simulink model "untitled2"  (R2016a)
settings: Solver=VariableStepAuto  StartTime=0.0  StopTime=500  FixedStep=0.01  RelTol=1e-3
undefined symbols (not defined in the file or in its folder): ref_speed
libraries: simulink x1
settings Model: Creator=91968  LastModifiedBy=91968

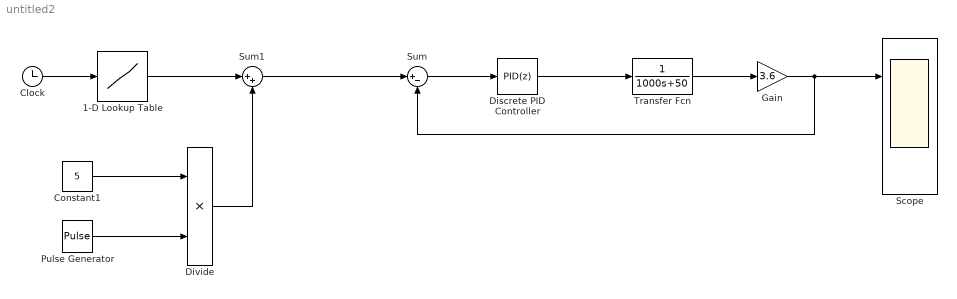
== system untitled2 ==
  1-D Lookup Table : Lookup_n-D  NumberOfTableDimensions=1  BreakpointsForDimension1=[-5:5]  Table=ref_speed(1:500)  InternalRulePriority=Speed  RndMeth=Simplest  InputSameDT=on
  Clock : Clock
  Constant1 : Constant  Value=5  VectorParams1D=off
  Discrete PID Controller : simulink/Continuous/PID Controller  Controller=PID  TimeDomain=Discrete-time  SampleTime=1  IntegratorMethod=Forward Euler  FilterMethod=Forward Euler  Form=Parallel  UseFilter=on  ControllerParametersSource=internal  P=200  I=7.1  D=0  N=100  InitialConditionSource=internal  InitialConditionForIntegrator=0  InitialConditionForFilter=0  ExternalReset=none  LimitOutput=on  UpperSaturationLimit=4200  LowerSaturationLimit=-inf  LinearizeAsGain=off  AntiWindupMode=none  Kb=1  TrackingMode=off  Kt=1  PParamMin=[]  PParamMax=[]  IParamMin=[]  IParamMax=[]  DParamMin=[]  DParamMax=[]  NParamMin=[]  NParamMax=[]  KbParamMin=[]  KbParamMax=[]  KtParamMin=[]  KtParamMax=[]  POutMin=[]  POutMax=[]  IOutMin=[]  IOutMax=[]  DOutMin=[]  DOutMax=[]  NOutMin=[]  NOutMax=[]  KbOutMin=[]  KbOutMax=[]  KtOutMin=[]  KtOutMax=[]  IntegratorOutMin=[]  IntegratorOutMax=[]  FilterOutMin=[]  FilterOutMax=[]  SumOutMin=[]  SumOutMax=[]  SumI1OutMin=[]  SumI1OutMax=[]  SumI2OutMin=[]  SumI2OutMax=[]  SumI3OutMin=[]  SumI3OutMax=[]  SumDOutMin=[]  SumDOutMax=[]  SaturationOutMin=[]  SaturationOutMax=[]  IntegratorContinuousStateAttributes=''  IntegratorStateMustResolveToSignalObject=off  IntegratorRTWStateStorageClass=Auto  FilterContinuousStateAttributes=''  FilterStateMustResolveToSignalObject=off  FilterRTWStateStorageClass=Auto  DifferentiatorICPrevScaledInput=0  DifferentiatorOutMin=[]  DifferentiatorOutMax=[]
  Divide : Product  Inputs=**
  Gain : Gain  Gain=3.6
  Pulse Generator : DiscretePulseGenerator  PulseType=Time based  Period=50
  Scope : Scope  NumInputPorts=2
  Sum : Sum  Inputs=|+-
  Sum1 : Sum  Inputs=|++
  Transfer Fcn : TransferFcn  Denominator=[1000 50]
  wires:
  Discrete PID Controller/1 -> Transfer Fcn/1
  1-D Lookup Table/1 -> Sum1/1
  Transfer Fcn/1 -> Gain/1
  Gain/1 -> Sum/2, Scope/1
  Sum/1 -> Discrete PID Controller/1
  Pulse Generator/1 -> Divide/2
  Sum1/1 -> Sum/1
  Constant1/1 -> Divide/1
  Divide/1 -> Sum1/2
  Clock/1 -> 1-D Lookup Table/1
